simulink model "Formation_FMS2"  (R2022b)
settings: Solver=FixedStepDiscrete  StartTime=0.0  StopTime=10.0  FixedStep=FMS_CONST.dt  RelTol=1e-3
values from neighbouring files (symbols this model uses):
  FMS_PARAM = Simulink.Parameter(FMS_PARAM_VALUE)    [fms_model_init.m]
  FORMATION_PARAM = Simulink.Parameter(FORMATION_PARAM_VALUE)    [fms_model_init.m]
undefined symbols (not defined in the file or in its folder): ax_cmd, ay_cmd, CONTROL_PARAM, DiscIntNeverNeededParam, PilotMode, state, VehicleState, vh_cmd
libraries: FC_Lib x51, simulink x16
(part 1 of 3)
settings Model: Creator=19114  LastModifiedBy=19114
settings OptimizationCC: DefaultParameterBehavior=Inlined  DefaultUnderspecifiedDataType=single  EnhancedBackFolding=on  PassReuseOutputArgsAs=Individual arguments  ZeroExternalMemoryAtStartup=off  ZeroInternalMemoryAtStartup=off  MaxStackSize=64  OptimizeBlockOrder=speed  DifferentSizesBufferReuse=on  OptimizationCustomize=off  EfficientTunableParamExpr=on
settings DebuggingCC: ParameterTunabilityLossMsg=error
settings HardwareCC: ProdBitPerLong=64  ProdHWDeviceType=Intel->x86-64 (Linux 64)
settings SFSimCC: MATLABDynamicMemAlloc=off
settings RTWCC: Description=Embedded Coder  SystemTargetFile=ert.tlc  PackageGeneratedCodeAndArtifacts=on  TemplateMakefile=ert_default_tmf  TargetLang=C++
settings CodeAppCC: ForceParamTrailComments=on  IgnoreCustomStorageClasses=off  OperatorAnnotations=on  SimulinkDataObjDesc=on  SFDataObjDesc=on  InsertBlockDesc=on
settings ERTTargetCC: TargetLangStandard=C++11 (ISO)  CodeInterfacePackaging=C++ class  SupportVariableSizeSignals=on  InlinedParameterPlacement=NonHierarchical  RootIOFormat=Structure reference  ERTCustomFileTemplate=example_file_process.tlc

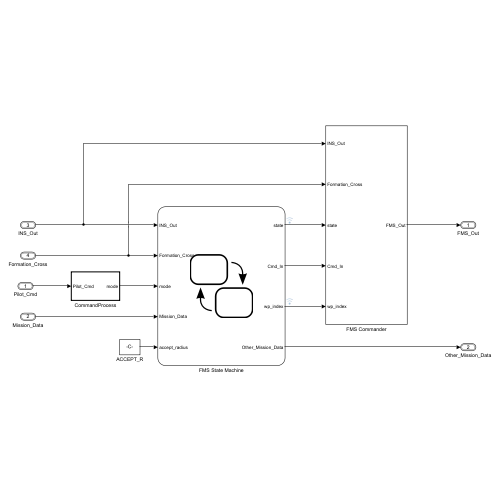
[thumbnail: Simulink's stored preview of the top-level diagram]
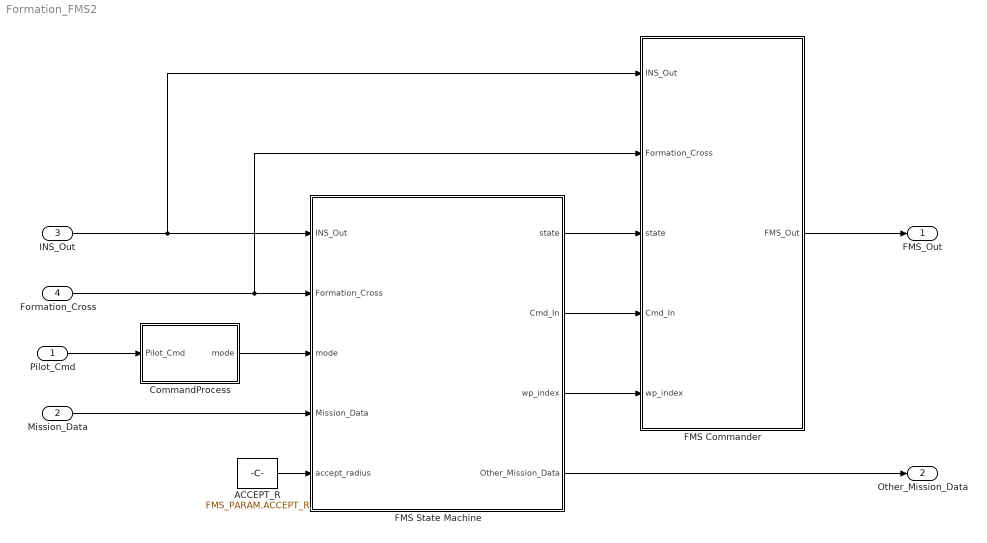
== system Formation_FMS2 ==
  Pilot_Cmd : Inport  OutDataTypeStr=Bus: Pilot_Cmd_Bus
  Mission_Data : Inport  Port=2  OutDataTypeStr=Bus: Mission_Data_Bus
  INS_Out : Inport  Port=3  OutDataTypeStr=Bus: INS_Out_Bus
  Formation_Cross : Inport  Port=4  OutDataTypeStr=Bus: Formation_Cross_Bus
  ACCEPT_R : Constant  Value=FMS_PARAM.ACCEPT_R
  CommandProcess : Subsystem  TreatAsAtomicUnit=on
  FMS Commander : Subsystem  mask{uav_id=3}
      mask DialogControl ParameterGroupVar Prompt: 参数
  FMS State Machine : Stateflow chart  TreatAsAtomicUnit=on  mask{uav_id=3, form_radius=FORMATION_PARAM.FORM_RADIUS}
  FMS_Out : Outport  OutDataTypeStr=Bus: FMS_Out_Bus  VectorParamsAs1DForOutWhenUnconnected=off
  Other_Mission_Data : Outport  Port=2  OutDataTypeStr=Bus: Other_Mission_Data_Bus  VectorParamsAs1DForOutWhenUnconnected=off
  wires:
  FMS State Machine/2(Cmd_In) -> FMS Commander/4(Cmd_In)
  ACCEPT_R/1 -> FMS State Machine/5(accept_radius)
  FMS State Machine/4(Other_Mission_Data) -> Other_Mission_Data/1
  Mission_Data/1 -> FMS State Machine/4(Mission_Data)
  Formation_Cross/1 -> FMS Commander/2(Formation_Cross), FMS State Machine/2(Formation_Cross)
  FMS State Machine/1(state) -> FMS Commander/3(state)
  CommandProcess/1(mode) -> FMS State Machine/3(mode)
  FMS Commander/1(FMS_Out) -> FMS_Out/1
  Pilot_Cmd/1 -> CommandProcess/1(Pilot_Cmd)
  FMS State Machine/3(wp_index) -> FMS Commander/5(wp_index)
  INS_Out/1 -> FMS Commander/1(INS_Out), FMS State Machine/1(INS_Out)

== system Formation_FMS2/CommandProcess ==
  Pilot_Cmd : Inport
  Check Valid : Subsystem
  Mode PreProcess : Subsystem
  mode : Outport  VectorParamsAs1DForOutWhenUnconnected=off
  wires:
  Pilot_Cmd/1 -> Check Valid/1(Pilot_Cmd), Mode PreProcess/2(Pilot_Cmd)
  Check Valid/1(pilot_cmd_valid) -> Mode PreProcess/1(pilot_cmd_valid)
  Mode PreProcess/1(mode) -> mode/1  "fms_mode"

== system Formation_FMS2/FMS Commander ==
  INS_Out : Inport
  Formation_Cross : Inport  Port=2
  state : Inport  Port=3
  Cmd_In : Inport  Port=4
  wp_index : Inport  Port=5
  Bus Creator : Subsystem
  Commander : Subsystem
  FMS_Out : Outport
  wires:
  INS_Out/1 -> Bus Creator/1(INS_Out)
  state/1 -> Bus Creator/3(state)
  Cmd_In/1 -> Bus Creator/4(Cmd_In)
  wp_index/1 -> Bus Creator/5(wp_index)
  Bus Creator/1(FMS_In) -> Commander/1(FMS_In)
  Commander/1(FMS_Out) -> FMS_Out/1
  Formation_Cross/1 -> Bus Creator/2(Formation_Cross)

== system Formation_FMS2/FMS State Machine/Vehicle.Formation.FormAssemble.dubinsPath ==
  Formation_Cross : Inport  OutDataTypeStr=Bus: Formation_Cross_Bus  PortDimensions=1
  f : TriggerPort  TriggerType=function-call  VariantControl=(inherit)
      settings: CopyFcn=Stateflow.SLINSF.SimulinkMan.removeBlockPreDeleteFcn  PreDeleteFcn=Stateflow.SLINSF.SimulinkMan.unsafePredeleteFcn
  MATLAB Function : MATLAB Function  TreatAsAtomicUnit=on  mask{form_points=FORMATION_PARAM.FORM_POINT}
  Other_Mission_Data : Outport  OutDataTypeStr=Bus: Other_Mission_Data_Bus  PortDimensions=1
  wires:
  Formation_Cross/1 -> MATLAB Function/1(ins)
  MATLAB Function/1(mission) -> Other_Mission_Data/1

== system Formation_FMS2/FMS State Machine/Vehicle.Formation.FormAssemble.dubinsPathRatio ==
  waypoints : Inport  OutDataTypeStr=single  PortDimensions=[5 5]
  pose : Inport  Port=2  OutDataTypeStr=single  PortDimensions=[1 3]
  wp_index : Inport  Port=3  OutDataTypeStr=uint16  PortDimensions=1
  f : TriggerPort  TriggerType=function-call  VariantControl=(inherit)
      settings: CopyFcn=Stateflow.SLINSF.SimulinkMan.removeBlockPreDeleteFcn  PreDeleteFcn=Stateflow.SLINSF.SimulinkMan.unsafePredeleteFcn
  Dubins Closest Point : FC_Lib/Fromation/Dubins Closest Point
      settings: LibrarySourceBlock=|
      | simulink/User-Defined
      | Functions/MATLAB Function
  Terminator : Terminator
  path_ratio : Outport  OutDataTypeStr=single  PortDimensions=1
  wires:
  Dubins Closest Point/1 -> path_ratio/1
  pose/1 -> Dubins Closest Point/2
  wp_index/1 -> Dubins Closest Point/3
  waypoints/1 -> Dubins Closest Point/1
  Dubins Closest Point/2 -> Terminator/1

== system Formation_FMS2/FMS State Machine/Vehicle.Formation.FormAssemble.testinf ==
  Input : Inport  OutDataTypeStr=single  PortDimensions=1
  f : TriggerPort  TriggerType=function-call  VariantControl=(inherit)
      settings: CopyFcn=Stateflow.SLINSF.SimulinkMan.removeBlockPreDeleteFcn  PreDeleteFcn=Stateflow.SLINSF.SimulinkMan.unsafePredeleteFcn
  MATLAB Function : MATLAB Function  TreatAsAtomicUnit=on
  Output : Outport  OutDataTypeStr=single  PortDimensions=1
  wires:
  Input/1 -> MATLAB Function/1(u)
  MATLAB Function/1(y) -> Output/1

== system Formation_FMS2/FMS State Machine/Vehicle.Formation.check_form_valid ==
  Formation_Cross : Inport  OutDataTypeStr=Bus: Formation_Cross_Bus  PortDimensions=1
  INS_Out : Inport  Port=2  OutDataTypeStr=Bus: INS_Out_Bus  PortDimensions=1
  f : TriggerPort  TriggerType=function-call  VariantControl=(inherit)
      settings: CopyFcn=Stateflow.SLINSF.SimulinkMan.removeBlockPreDeleteFcn  PreDeleteFcn=Stateflow.SLINSF.SimulinkMan.unsafePredeleteFcn
  MATLAB Function : MATLAB Function  TreatAsAtomicUnit=on  mask{form_radius=form_radius}
  valid : Outport  OutDataTypeStr=uint32  PortDimensions=1
  wires:
  Formation_Cross/1 -> MATLAB Function/1(Formation_Cross)
  INS_Out/1 -> MATLAB Function/2(INS_Out)
  MATLAB Function/1(valid) -> valid/1

== system Formation_FMS2/CommandProcess/Check Valid ==
  Pilot_Cmd : Inport
  Bus Selector1 : BusSelector  OutputSignals=timestamp
  Compare To Constant1 : simulink/Logic and Bit Operations/Compare To Constant  relop=<  const=0.5  OutDataTypeStr=boolean
  Constant1 : Constant  OutDataTypeStr=single
  Detect Change1 : simulink/Logic and Bit Operations/Detect Change  vinit=0  OutDataTypeStr=boolean
  Discrete-Time Integrator1 : DiscreteIntegrator  ExternalReset=sampled level  SampleTime=-1  SaturateOnIntegerOverflow=on  ICPrevOutput=DiscIntNeverNeededParam  ICPrevScaledInput=DiscIntNeverNeededParam
  pilot_cmd_valid : Outport  VectorParamsAs1DForOutWhenUnconnected=off
  wires:
  Pilot_Cmd/1 -> Bus Selector1/1
  Compare To Constant1/1 -> pilot_cmd_valid/1
  Bus Selector1/1 -> Detect Change1/1  "<timestamp>"
  Constant1/1 -> Discrete-Time Integrator1/1
  Detect Change1/1 -> Discrete-Time Integrator1/2
  Discrete-Time Integrator1/1 -> Compare To Constant1/1

== system Formation_FMS2/CommandProcess/Mode PreProcess ==
  pilot_cmd_valid : Inport
  Pilot_Cmd : Inport  Port=2
  Bus Selector1 : BusSelector  OutputSignals=mode
  Compare To Zero1 : simulink/Logic and Bit Operations/Compare To Zero  relop=~=  OutDataTypeStr=boolean
  Data Type Conversion2 : DataTypeConversion  OutDataTypeStr=Enum: PilotMode  SaturateOnIntegerOverflow=off  RndMeth=Floor
  Delay : Delay  DelayLength=1  InitialCondition=PilotMode.None
  Logical Operator1 : Logic  AllPortsSameDT=off  OutDataTypeStr=boolean
  Switch : Switch  Criteria=u2 > Threshold  SaturateOnIntegerOverflow=off  InputSameDT=off
  mode : Outport  VectorParamsAs1DForOutWhenUnconnected=off
  wires:
  Pilot_Cmd/1 -> Bus Selector1/1
  Bus Selector1/1 -> Compare To Zero1/1, Data Type Conversion2/1  "<mode>"
  Logical Operator1/1 -> Switch/2
  Data Type Conversion2/1 -> Switch/1
  Switch/1 -> mode/1, Delay/1
  Delay/1 -> Switch/3
  pilot_cmd_valid/1 -> Logical Operator1/2
  Compare To Zero1/1 -> Logical Operator1/1

== system Formation_FMS2/FMS Commander/Bus Creator ==
  INS_Out : Inport
  Formation_Cross : Inport  Port=2
  state : Inport  Port=3
  Cmd_In : Inport  Port=4
  wp_index : Inport  Port=5
  Bus Creator : BusCreator  Inputs=5
  Signal Copy{1..3,5..6} (5 alike) : SignalConversion  OverrideOpt=off
  FMS_In : Outport
  wires:
  Bus Creator/1 -> FMS_In/1
  wp_index/1 -> Signal Copy5/1
  Signal Copy3/1 -> Bus Creator/4  "Cmd_In"
  Signal Copy1/1 -> Bus Creator/1  "INS_Out"
  INS_Out/1 -> Signal Copy1/1
  Signal Copy5/1 -> Bus Creator/5  "wp_index"
  Signal Copy6/1 -> Bus Creator/3  "vehicle_state"
  state/1 -> Signal Copy6/1
  Cmd_In/1 -> Signal Copy3/1
  Formation_Cross/1 -> Signal Copy2/1
  Signal Copy2/1 -> Bus Creator/2  "Formation_Cross"

== system Formation_FMS2/FMS Commander/Commander ==
  FMS_In : Inport
  Bus Selector : BusSelector  OutputSignals=vehicle_state
  Default : Subsystem
      settings: UndoDeleteFcn=Stateflow.SLINSF.SimulinkMan.restorePreDeleteFcn  PreDeleteFcn=Stateflow.SLINSF.SimulinkMan.removePreDeleteFcn
  FMS_In1 : InportShadow
  FMS_In2 : InportShadow
  FMS_In3 : InportShadow
  Form_Subsystem : Subsystem  TreatAsAtomicUnit=on
  Hold : Subsystem
      settings: UndoDeleteFcn=Stateflow.SLINSF.SimulinkMan.restorePreDeleteFcn  PreDeleteFcn=Stateflow.SLINSF.SimulinkMan.removePreDeleteFcn
  Merge : Merge  Inputs=3
  Switch Case : SwitchCase  CaseConditions={[VehicleState.FormAssemble,VehicleState.FormHold,VehicleState.FormMission,VehicleState.FormDisband],VehicleState.Hold}
  FMS_Out : Outport
  wires:
  FMS_In/1 -> Bus Selector/1
  Bus Selector/1 -> Switch Case/1  "<vehicle_state>"
  Switch Case/1 -> Form_Subsystem/Action
  FMS_In1/1 -> Form_Subsystem/1(FMS_In)
  Form_Subsystem/1(FMS_Out) -> Merge/1
  Merge/1 -> FMS_Out/1
  Switch Case/2 -> Hold/Action
  Hold/1(FMS_Out) -> Merge/2
  FMS_In2/1 -> Hold/1(FMS_In)
  Switch Case/3 -> Default/Action
  Default/1(FMS_Out) -> Merge/3
  FMS_In3/1 -> Default/1(FMS_In)

== system Formation_FMS2/FMS Commander/Commander/Default ==
  FMS_In : Inport
  Action Port : ActionPort  InitializeStates=reset
      settings: CopyFcn=Stateflow.SLINSF.SimulinkMan.removeBlockPreDeleteFcn
  Airspeed Hold : Subsystem
  Altitude_Hold : Subsystem
  Bus Assignment : BusAssignment  AssignedSignals=state,ax_cmd,ay_cmd,vh_cmd
  Constant : Constant  Value=0  OutDataTypeStr=Bus: FMS_Out_Bus
  Constant1 : Constant  Value=VehicleState.None  OutDataTypeStr=Enum: VehicleState
  Loiter_Control : Subsystem  Commented=on
  FMS_Out : Outport  VectorParamsAs1DForOutWhenUnconnected=off
  wires:
  Airspeed Hold/1(ax_cmd) -> Bus Assignment/3
  Loiter_Control/1(ay_cmd_mPs2) -> Bus Assignment/4
  FMS_In/1 -> Airspeed Hold/1(FMS_In), Altitude_Hold/1(FMS_In), Loiter_Control/1(FMS_In)
  Constant/1 -> Bus Assignment/1
  Altitude_Hold/1(vh_cmd_mPs) -> Bus Assignment/5
  Bus Assignment/1 -> FMS_Out/1
  Constant1/1 -> Bus Assignment/2

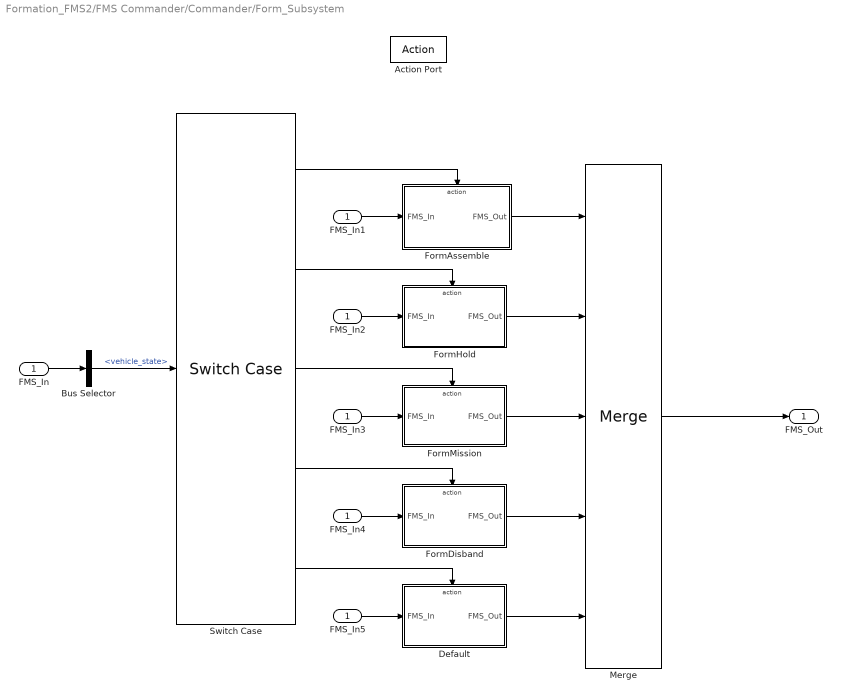
== system Formation_FMS2/FMS Commander/Commander/Form_Subsystem ==
  FMS_In : Inport
  Action Port : ActionPort
  Bus Selector : BusSelector  OutputSignals=vehicle_state
  Default : Subsystem
      settings: UndoDeleteFcn=Stateflow.SLINSF.SimulinkMan.restorePreDeleteFcn  PreDeleteFcn=Stateflow.SLINSF.SimulinkMan.removePreDeleteFcn
  FMS_In{1..5} (5 alike) : InportShadow
  FormAssemble : Subsystem  TreatAsAtomicUnit=on
  FormDisband : Subsystem
      settings: UndoDeleteFcn=Stateflow.SLINSF.SimulinkMan.restorePreDeleteFcn  PreDeleteFcn=Stateflow.SLINSF.SimulinkMan.removePreDeleteFcn
  FormHold : Subsystem
      settings: UndoDeleteFcn=Stateflow.SLINSF.SimulinkMan.restorePreDeleteFcn  PreDeleteFcn=Stateflow.SLINSF.SimulinkMan.removePreDeleteFcn
  FormMission : Subsystem  TreatAsAtomicUnit=on
  Merge : Merge  Inputs=5
  Switch Case : SwitchCase  CaseConditions={VehicleState.FormAssemble,VehicleState.FormHold,VehicleState.FormMission,VehicleState.FormDisband}
  FMS_Out : Outport
  wires:
  Merge/1 -> FMS_Out/1
  FMS_In/1 -> Bus Selector/1
  Bus Selector/1 -> Switch Case/1  "<vehicle_state>"
  Switch Case/5 -> Default/Action
  Default/1(FMS_Out) -> Merge/5
  Switch Case/3 -> FormMission/Action
  FMS_In1/1 -> FormAssemble/1(FMS_In)
  Switch Case/1 -> FormAssemble/Action
  FMS_In2/1 -> FormHold/1(FMS_In)
  Switch Case/2 -> FormHold/Action
  FMS_In3/1 -> FormMission/1(FMS_In)
  Switch Case/4 -> FormDisband/Action
  FMS_In4/1 -> FormDisband/1(FMS_In)
  FMS_In5/1 -> Default/1(FMS_In)
  FormAssemble/1(FMS_Out) -> Merge/1
  FormHold/1(FMS_Out) -> Merge/2
  FormMission/1(FMS_Out) -> Merge/3
  FormDisband/1(FMS_Out) -> Merge/4

== system Formation_FMS2/FMS Commander/Commander/Hold ==
  FMS_In : Inport
  Action Port : ActionPort  InitializeStates=reset
      settings: CopyFcn=Stateflow.SLINSF.SimulinkMan.removeBlockPreDeleteFcn
  Airspeed Hold : Subsystem
  Altitude_Hold : Subsystem
  Bus Assignment : BusAssignment  AssignedSignals=state,ax_cmd,ay_cmd,vh_cmd
  Constant : Constant  Value=0  OutDataTypeStr=Bus: FMS_Out_Bus
  Constant1 : Constant  Value=VehicleState.Hold  OutDataTypeStr=Enum: VehicleState
  Loiter_Control : Subsystem
  FMS_Out : Outport  VectorParamsAs1DForOutWhenUnconnected=off
  wires:
  Bus Assignment/1 -> FMS_Out/1
  Altitude_Hold/1(vh_cmd_mPs) -> Bus Assignment/5
  Constant/1 -> Bus Assignment/1
  FMS_In/1 -> Altitude_Hold/1(FMS_In), Airspeed Hold/1(FMS_In), Loiter_Control/1(FMS_In)
  Loiter_Control/1(ay_cmd_mPs2) -> Bus Assignment/4
  Airspeed Hold/1(ax_cmd) -> Bus Assignment/3
  Constant1/1 -> Bus Assignment/2

== system Formation_FMS2/FMS Commander/Commander/Default/Airspeed Hold ==
  FMS_In : Inport
  Bus Selector : BusSelector  OutputSignals=INS_Out.airspeed
  Constant : Constant  Value=FMS_PARAM.FW_AIRSPD_TRIM
  Gain : Gain
  Sum : Sum  Inputs=-+|
  ax_cmd : Outport
  wires:
  Bus Selector/1 -> Sum/1  "<airspeed>"
  FMS_In/1 -> Bus Selector/1
  Constant/1 -> Sum/2
  Gain/1 -> ax_cmd/1  "ax_cmd"
  Sum/1 -> Gain/1  "v_error"

== system Formation_FMS2/FMS Commander/Commander/Default/Altitude_Hold ==
  FMS_In : Inport
  Bus Selector2 : BusSelector  OutputSignals=INS_Out.h_R
  Delay : Delay  DelayLength=1  InitialConditionSource=Input port
      settings: InputPortMap=u0,p4
  Gain2 : Gain  Gain=FMS_PARAM.Z_P  OutDataTypeStr=single
  Saturation : Saturate  UpperLimit=CONTROL_PARAM.FW_T_CLMB_MAX  LowerLimit=-CONTROL_PARAM.FW_T_SINK_MAX
  Sum : Sum  Inputs=-+|
  vh_cmd_mPs : Outport  VectorParamsAs1DForOutWhenUnconnected=off
  wires:
  Gain2/1 -> Saturation/1
  Bus Selector2/1 -> Delay/2, Sum/1  "<h_R>"
  Sum/1 -> Gain2/1  "h_err_R"
  Delay/1 -> Sum/2, Delay/1  "h_cmd_R"
  FMS_In/1 -> Bus Selector2/1
  Saturation/1 -> vh_cmd_mPs/1

== system Formation_FMS2/FMS Commander/Commander/Default/Loiter_Control ==
  FMS_In : Inport
  Bus Selector2 : BusSelector  OutputSignals=INS_Out.vn,INS_Out.ve
  L1 : Constant  Value=FMS_PARAM.L1  OutDataTypeStr=single
  L1 Reference WP : Subsystem
  L1_Core : Subsystem
  Mux1 : Mux  Inputs=2
  R : Constant  Value=FMS_PARAM.LOITER_R  OutDataTypeStr=single
  Reference_Point : Subsystem
  ay_cmd_mPs2 : Outport  VectorParamsAs1DForOutWhenUnconnected=off
  wires:
  Mux1/1 -> L1_Core/4(Vg)
  Bus Selector2/1 -> Mux1/1  "<vn>"
  Bus Selector2/2 -> Mux1/2  "<ve>"
  FMS_In/1 -> Reference_Point/1(FMS_In), Bus Selector2/1
  L1/1 -> L1 Reference WP/5(L1), L1_Core/3(L1)
  R/1 -> L1 Reference WP/4(R)
  Reference_Point/3(n) -> L1 Reference WP/3(n)
  Reference_Point/2(p_0) -> L1 Reference WP/2(P_0)
  Reference_Point/1(p_vehicle) -> L1 Reference WP/1(P_Vehicle), L1_Core/1(p_vehicle)
  L1_Core/1(ay_cmd_mPs2) -> ay_cmd_mPs2/1
  L1 Reference WP/1(L1_WP) -> L1_Core/2(L1_WP)  "L1_WP"

== system Formation_FMS2/FMS Commander/Commander/Form_Subsystem/Default ==
  FMS_In : Inport
  Action Port : ActionPort  InitializeStates=reset
      settings: CopyFcn=Stateflow.SLINSF.SimulinkMan.removeBlockPreDeleteFcn
  Airspeed Hold : Subsystem
  Altitude_Hold : Subsystem
  Bus Assignment : BusAssignment  AssignedSignals=state,ax_cmd,ay_cmd,vh_cmd
  Constant : Constant  Value=0  OutDataTypeStr=Bus: FMS_Out_Bus
  Constant1 : Constant  Value=VehicleState.None  OutDataTypeStr=Enum: VehicleState
  Loiter_Control : Subsystem  Commented=on
  FMS_Out : Outport  VectorParamsAs1DForOutWhenUnconnected=off
  wires:
  Airspeed Hold/1(ax_cmd) -> Bus Assignment/3
  Loiter_Control/1(ay_cmd_mPs2) -> Bus Assignment/4
  FMS_In/1 -> Airspeed Hold/1(FMS_In), Altitude_Hold/1(FMS_In), Loiter_Control/1(FMS_In)
  Constant/1 -> Bus Assignment/1
  Altitude_Hold/1(vh_cmd_mPs) -> Bus Assignment/5
  Bus Assignment/1 -> FMS_Out/1
  Constant1/1 -> Bus Assignment/2

== system Formation_FMS2/FMS Commander/Commander/Form_Subsystem/FormAssemble ==
  FMS_In : Inport
  Action Port : ActionPort
  Bus Selector : BusSelector  OutputSignals=wp_index
  Detect Change : simulink/Logic and Bit Operations/Detect Change  vinit=0  OutDataTypeStr=boolean
  Mission_SubSystem : Subsystem  TreatAsAtomicUnit=on
  FMS_Out : Outport
  wires:
  FMS_In/1 -> Bus Selector/1, Mission_SubSystem/1(FMS_In)
  Mission_SubSystem/1(FMS_Out) -> FMS_Out/1
  Detect Change/1 -> Mission_SubSystem/Reset
  Bus Selector/1 -> Detect Change/1  "<wp_index>"

== system Formation_FMS2/FMS Commander/Commander/Form_Subsystem/FormDisband ==
  FMS_In : Inport
  Action Port : ActionPort  InitializeStates=reset
      settings: CopyFcn=Stateflow.SLINSF.SimulinkMan.removeBlockPreDeleteFcn
  Airspeed Hold : Subsystem
  Altitude_Hold : Subsystem
  Bus Assignment : BusAssignment  AssignedSignals=state,ax_cmd,ay_cmd,vh_cmd
  Constant : Constant  Value=0  OutDataTypeStr=Bus: FMS_Out_Bus
  Constant1 : Constant  Value=VehicleState.FormDisband  OutDataTypeStr=Enum: VehicleState
  Loiter_Control : Subsystem
  FMS_Out : Outport  VectorParamsAs1DForOutWhenUnconnected=off
  wires:
  Constant1/1 -> Bus Assignment/2
  Airspeed Hold/1(ax_cmd) -> Bus Assignment/3
  Loiter_Control/1(ay_cmd_mPs2) -> Bus Assignment/4
  FMS_In/1 -> Loiter_Control/1(FMS_In), Airspeed Hold/1(FMS_In), Altitude_Hold/1(FMS_In)
  Constant/1 -> Bus Assignment/1
  Altitude_Hold/1(vh_cmd_mPs) -> Bus Assignment/5
  Bus Assignment/1 -> FMS_Out/1

== system Formation_FMS2/FMS Commander/Commander/Form_Subsystem/FormHold ==
  FMS_In : Inport
  Action Port : ActionPort  InitializeStates=reset
      settings: CopyFcn=Stateflow.SLINSF.SimulinkMan.removeBlockPreDeleteFcn
  Airspeed Hold : Subsystem
  Altitude_Hold : Subsystem
  Bus Assignment : BusAssignment  AssignedSignals=state,ax_cmd,ay_cmd,vh_cmd
  Constant : Constant  Value=0  OutDataTypeStr=Bus: FMS_Out_Bus
  Constant1 : Constant  Value=VehicleState.FormHold  OutDataTypeStr=Enum: VehicleState
  Loiter_Control : Subsystem
  FMS_Out : Outport  VectorParamsAs1DForOutWhenUnconnected=off
  wires:
  Bus Assignment/1 -> FMS_Out/1
  Altitude_Hold/1(vh_cmd_mPs) -> Bus Assignment/5
  Constant/1 -> Bus Assignment/1
  FMS_In/1 -> Altitude_Hold/1(FMS_In), Airspeed Hold/1(FMS_In), Loiter_Control/1(FMS_In)
  Loiter_Control/1(ay_cmd_mPs2) -> Bus Assignment/4
  Airspeed Hold/1(ax_cmd) -> Bus Assignment/3
  Constant1/1 -> Bus Assignment/2

== system Formation_FMS2/FMS Commander/Commander/Form_Subsystem/FormMission ==
  FMS_In : Inport
  Action Port : ActionPort
  Bus Selector : BusSelector  OutputSignals=wp_index
  Detect Change : simulink/Logic and Bit Operations/Detect Change  vinit=0  OutDataTypeStr=boolean
  FormMission_SubSystem : Subsystem  TreatAsAtomicUnit=on
  FMS_Out : Outport
  wires:
  FMS_In/1 -> Bus Selector/1, FormMission_SubSystem/1(FMS_In)
  FormMission_SubSystem/1(FMS_Out) -> FMS_Out/1
  Detect Change/1 -> FormMission_SubSystem/Reset
  Bus Selector/1 -> Detect Change/1  "<wp_index>"

== system Formation_FMS2/FMS Commander/Commander/Hold/Airspeed Hold ==
  FMS_In : Inport
  Bus Selector : BusSelector  OutputSignals=INS_Out.airspeed
  Constant : Constant  Value=FMS_PARAM.FW_AIRSPD_TRIM
  Gain : Gain
  Sum : Sum  Inputs=-+|
  ax_cmd : Outport
  wires:
  Sum/1 -> Gain/1  "v_error"
  Gain/1 -> ax_cmd/1  "ax_cmd"
  Constant/1 -> Sum/2
  FMS_In/1 -> Bus Selector/1
  Bus Selector/1 -> Sum/1  "<airspeed>"

== system Formation_FMS2/FMS Commander/Commander/Hold/Altitude_Hold ==
  FMS_In : Inport
  Bus Selector2 : BusSelector  OutputSignals=INS_Out.h_R
  Constant : Constant  Value=FMS_PARAM.FW_HEIGHT_TRIM
  Delay : Delay  DelayLength=1  InitialConditionSource=Input port
      settings: InputPortMap=u0,p4
  Gain2 : Gain  Gain=FMS_PARAM.Z_P  OutDataTypeStr=single
  Saturation : Saturate  UpperLimit=CONTROL_PARAM.FW_T_CLMB_MAX  LowerLimit=-CONTROL_PARAM.FW_T_SINK_MAX
  Sum : Sum  Inputs=-+|
  vh_cmd_mPs : Outport  VectorParamsAs1DForOutWhenUnconnected=off
  wires:
  Gain2/1 -> Saturation/1
  Bus Selector2/1 -> Sum/1  "<h_R>"
  Sum/1 -> Gain2/1  "h_err_R"
  Delay/1 -> Sum/2, Delay/1  "h_cmd_R"
  FMS_In/1 -> Bus Selector2/1
  Saturation/1 -> vh_cmd_mPs/1
  Constant/1 -> Delay/2

== system Formation_FMS2/FMS Commander/Commander/Hold/Loiter_Control ==
  FMS_In : Inport
  Bus Selector2 : BusSelector  OutputSignals=INS_Out.vn,INS_Out.ve
  L1 : Constant  Value=FMS_PARAM.L1  OutDataTypeStr=single
  L1 Reference WP : Subsystem
  L1_Core : Subsystem
  Mux1 : Mux  Inputs=2
  R : Constant  Value=FMS_PARAM.LOITER_R  OutDataTypeStr=single
  Reference_Point : Subsystem
  ay_cmd_mPs2 : Outport  VectorParamsAs1DForOutWhenUnconnected=off
  wires:
  L1 Reference WP/1(L1_WP) -> L1_Core/2(L1_WP)  "L1_WP"
  L1_Core/1(ay_cmd_mPs2) -> ay_cmd_mPs2/1
  Reference_Point/1(p_vehicle) -> L1_Core/1(p_vehicle), L1 Reference WP/1(P_Vehicle)
  Reference_Point/2(p_0) -> L1 Reference WP/2(P_0)
  Reference_Point/3(n) -> L1 Reference WP/3(n)
  R/1 -> L1 Reference WP/4(R)
  L1/1 -> L1_Core/3(L1), L1 Reference WP/5(L1)
  FMS_In/1 -> Bus Selector2/1, Reference_Point/1(FMS_In)
  Bus Selector2/2 -> Mux1/2  "<ve>"
  Bus Selector2/1 -> Mux1/1  "<vn>"
  Mux1/1 -> L1_Core/4(Vg)

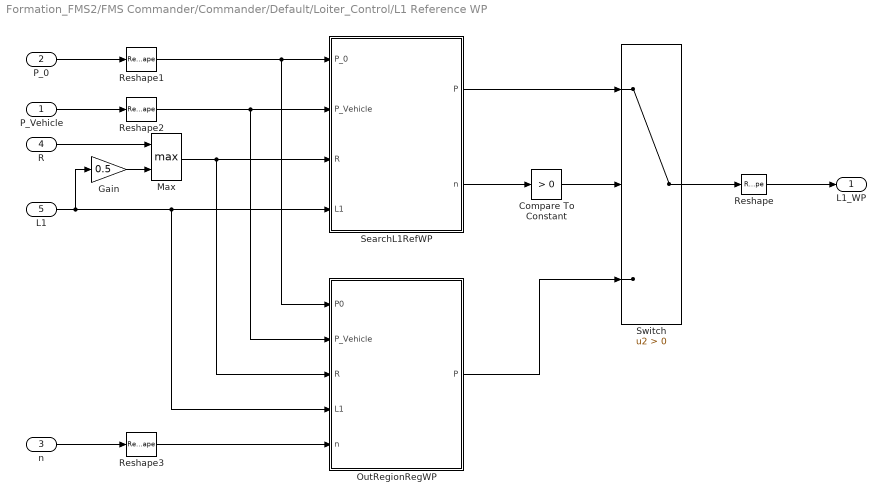
== system Formation_FMS2/FMS Commander/Commander/Default/Loiter_Control/L1 Reference WP ==
  P_Vehicle : Inport
  P_0 : Inport  Port=2
  n : Inport  Port=3
  R : Inport  Port=4
  L1 : Inport  Port=5
  Compare To Constant : simulink/Logic and Bit Operations/Compare To Constant  relop=>  const=0  OutDataTypeStr=boolean
  Gain : Gain  Gain=0.5
  Max : MinMax  Function=max  Inputs=2
  OutRegionRegWP : MATLAB Function  TreatAsAtomicUnit=on
  Reshape : Reshape  OutputDimensionality=Customize  OutputDimensions=[2,1]
  Reshape1 : Reshape  OutputDimensionality=Column vector (2-D)
  Reshape2 : Reshape  OutputDimensionality=Column vector (2-D)
  Reshape3 : Reshape  OutputDimensionality=Column vector (2-D)
  SearchL1RefWP : MATLAB Function  TreatAsAtomicUnit=on
  Switch : Switch  Criteria=u2 > Threshold  SaturateOnIntegerOverflow=off  InputSameDT=off
  L1_WP : Outport  VectorParamsAs1DForOutWhenUnconnected=off
  wires:
  Gain/1 -> Max/2
  R/1 -> Max/1
  Reshape3/1 -> OutRegionRegWP/5(n)
  n/1 -> Reshape3/1
  Reshape2/1 -> SearchL1RefWP/2(P_Vehicle), OutRegionRegWP/2(P_Vehicle)
  Reshape1/1 -> SearchL1RefWP/1(P_0), OutRegionRegWP/1(P0)
  L1/1 -> SearchL1RefWP/4(L1), OutRegionRegWP/4(L1), Gain/1
  Max/1 -> SearchL1RefWP/3(R), OutRegionRegWP/3(R)
  P_Vehicle/1 -> Reshape2/1
  P_0/1 -> Reshape1/1
  SearchL1RefWP/1(P) -> Switch/1
  Switch/1 -> Reshape/1
  OutRegionRegWP/1(P) -> Switch/3
  SearchL1RefWP/2(n) -> Compare To Constant/1
  Compare To Constant/1 -> Switch/2
  Reshape/1 -> L1_WP/1

== system Formation_FMS2/FMS Commander/Commander/Default/Loiter_Control/L1_Core ==
  p_vehicle : Inport
  L1_WP : Inport  Port=2
  L1 : Inport  Port=3
  Vg : Inport  Port=4
  L1_Lateral_Acceleration : Subsystem
  Subtract : Sum  Inputs=+-
  ay_cmd_mPs2 : Outport  VectorParamsAs1DForOutWhenUnconnected=off
  wires:
  L1_Lateral_Acceleration/1(l1_a_cmd) -> ay_cmd_mPs2/1
  Subtract/1 -> L1_Lateral_Acceleration/3(l1_path)
  Vg/1 -> L1_Lateral_Acceleration/2(Vg)
  L1/1 -> L1_Lateral_Acceleration/1(L1)
  p_vehicle/1 -> Subtract/2
  L1_WP/1 -> Subtract/1

== system Formation_FMS2/FMS Commander/Commander/Default/Loiter_Control/Reference_Point ==
  FMS_In : Inport
  Bus Selector1 : BusSelector  OutputSignals=Cmd_In.cur_waypoint
  Bus Selector2 : BusSelector  OutputSignals=INS_Out.vn,INS_Out.ve
  Bus Selector3 : BusSelector  OutputSignals=INS_Out.x_R,INS_Out.y_R
  Mux1 : Mux  Inputs=2
  Mux2 : Mux  Inputs=2
  Selector : Selector  InputPortWidth=3  IndexOptions=Index vector (dialog)  Indices=[1 2]  OutputSizes=1
  Vector Normalize : FC_Lib/Math/Vector Normalize
      settings: SourceProductName=Flight Control Toolbox
  start_vel : Delay  DelayLength=1  InitialConditionSource=Input port
      settings: InputPortMap=u0,p4
  p_vehicle : Outport  VectorParamsAs1DForOutWhenUnconnected=off
  p_0 : Outport  Port=2  VectorParamsAs1DForOutWhenUnconnected=off
  n : Outport  Port=3  VectorParamsAs1DForOutWhenUnconnected=off
  wires:
  Selector/1 -> p_0/1
  Bus Selector1/1 -> Selector/1  "<cur_waypoint>"
  Mux2/1 -> p_vehicle/1
  Bus Selector3/2 -> Mux2/2  "<y_R>"
  Bus Selector3/1 -> Mux2/1  "<x_R>"
  Mux1/1 -> start_vel/2
  FMS_In/1 -> Bus Selector1/1, Bus Selector2/1, Bus Selector3/1
  Vector Normalize/1 -> n/1
  Bus Selector2/1 -> Mux1/1  "<vn>"
  start_vel/1 -> start_vel/1, Vector Normalize/1
  Bus Selector2/2 -> Mux1/2  "<ve>"

== system Formation_FMS2/FMS Commander/Commander/Form_Subsystem/Default/Airspeed Hold ==
  FMS_In : Inport
  Bus Selector : BusSelector  OutputSignals=INS_Out.airspeed
  Constant : Constant  Value=FMS_PARAM.FW_AIRSPD_TRIM
  Gain : Gain
  Sum : Sum  Inputs=-+|
  ax_cmd : Outport
  wires:
  Bus Selector/1 -> Sum/1  "<airspeed>"
  FMS_In/1 -> Bus Selector/1
  Constant/1 -> Sum/2
  Gain/1 -> ax_cmd/1  "ax_cmd"
  Sum/1 -> Gain/1  "v_error"

== system Formation_FMS2/FMS Commander/Commander/Form_Subsystem/Default/Altitude_Hold ==
  FMS_In : Inport
  Bus Selector2 : BusSelector  OutputSignals=INS_Out.h_R
  Delay : Delay  DelayLength=1  InitialConditionSource=Input port
      settings: InputPortMap=u0,p4
  Gain2 : Gain  Gain=FMS_PARAM.Z_P  OutDataTypeStr=single
  Saturation : Saturate  UpperLimit=CONTROL_PARAM.FW_T_CLMB_MAX  LowerLimit=-CONTROL_PARAM.FW_T_SINK_MAX
  Sum : Sum  Inputs=-+|
  vh_cmd_mPs : Outport  VectorParamsAs1DForOutWhenUnconnected=off
  wires:
  Gain2/1 -> Saturation/1
  Bus Selector2/1 -> Delay/2, Sum/1  "<h_R>"
  Sum/1 -> Gain2/1  "h_err_R"
  Delay/1 -> Sum/2, Delay/1  "h_cmd_R"
  FMS_In/1 -> Bus Selector2/1
  Saturation/1 -> vh_cmd_mPs/1

== system Formation_FMS2/FMS Commander/Commander/Form_Subsystem/Default/Loiter_Control ==
  FMS_In : Inport
  Bus Selector2 : BusSelector  OutputSignals=INS_Out.vn,INS_Out.ve
  L1 : Constant  Value=FMS_PARAM.L1  OutDataTypeStr=single
  L1 Reference WP : Subsystem
  L1_Core : Subsystem
  Mux1 : Mux  Inputs=2
  R : Constant  Value=FMS_PARAM.LOITER_R  OutDataTypeStr=single
  Reference_Point : Subsystem
  ay_cmd_mPs2 : Outport  VectorParamsAs1DForOutWhenUnconnected=off
  wires:
  Mux1/1 -> L1_Core/4(Vg)
  Bus Selector2/1 -> Mux1/1  "<vn>"
  Bus Selector2/2 -> Mux1/2  "<ve>"
  FMS_In/1 -> Reference_Point/1(FMS_In), Bus Selector2/1
  L1/1 -> L1 Reference WP/5(L1), L1_Core/3(L1)
  R/1 -> L1 Reference WP/4(R)
  Reference_Point/3(n) -> L1 Reference WP/3(n)
  Reference_Point/2(p_0) -> L1 Reference WP/2(P_0)
  Reference_Point/1(p_vehicle) -> L1 Reference WP/1(P_Vehicle), L1_Core/1(p_vehicle)
  L1_Core/1(ay_cmd_mPs2) -> ay_cmd_mPs2/1
  L1 Reference WP/1(L1_WP) -> L1_Core/2(L1_WP)  "L1_WP"

== system Formation_FMS2/FMS Commander/Commander/Form_Subsystem/FormAssemble/Mission_SubSystem ==
  FMS_In : Inport
  Reset : ResetPort  DisableCoverage=on
  Airspeed Hold : Subsystem
  Altitude Control : Subsystem  Commented=on
  Altitude_Hold : Subsystem
  Bus Assignment : BusAssignment  AssignedSignals=state,ax_cmd,ay_cmd,vh_cmd
  Constant : Constant  Value=0  OutDataTypeStr=Bus: FMS_Out_Bus
  Constant1 : Constant  Value=VehicleState.FormAssemble  OutDataTypeStr=Enum: VehicleState
  Position Command : Subsystem
  testnan : MATLAB Function  Commented=on  TreatAsAtomicUnit=on
  FMS_Out : Outport  VectorParamsAs1DForOutWhenUnconnected=off
  wires:
  Constant/1 -> Bus Assignment/1
  Bus Assignment/1 -> FMS_Out/1
  Position Command/1(ay_cmd_mPs2) -> Bus Assignment/4
  Altitude_Hold/1(vh_cmd_mPs) -> Bus Assignment/5
  Airspeed Hold/1(ax_cmd) -> Bus Assignment/3
  Constant1/1 -> Bus Assignment/2
  FMS_In/1 -> Airspeed Hold/1(FMS_In), Position Command/1(FMS_In), Altitude_Hold/1(FMS_In)

== system Formation_FMS2/FMS Commander/Commander/Form_Subsystem/FormDisband/Airspeed Hold ==
  FMS_In : Inport
  Bus Selector : BusSelector  OutputSignals=INS_Out.airspeed
  Constant : Constant  Value=FMS_PARAM.FW_AIRSPD_TRIM
  Gain : Gain
  Sum : Sum  Inputs=-+|
  ax_cmd : Outport
  wires:
  Bus Selector/1 -> Sum/1  "<airspeed>"
  FMS_In/1 -> Bus Selector/1
  Constant/1 -> Sum/2
  Gain/1 -> ax_cmd/1  "ax_cmd"
  Sum/1 -> Gain/1  "v_error"

== system Formation_FMS2/FMS Commander/Commander/Form_Subsystem/FormDisband/Altitude_Hold ==
  FMS_In : Inport
  Bus Selector2 : BusSelector  OutputSignals=INS_Out.h_R
  Constant : Constant  Value=FMS_PARAM.FW_HEIGHT_TRIM
  Delay : Delay  DelayLength=1  InitialConditionSource=Input port
      settings: InputPortMap=u0,p4
  Gain2 : Gain  Gain=FMS_PARAM.Z_P  OutDataTypeStr=single
  Saturation : Saturate  UpperLimit=CONTROL_PARAM.FW_T_CLMB_MAX  LowerLimit=-CONTROL_PARAM.FW_T_SINK_MAX
  Sum : Sum  Inputs=-+|
  vh_cmd_mPs : Outport  VectorParamsAs1DForOutWhenUnconnected=off
  wires:
  Constant/1 -> Delay/2
  Saturation/1 -> vh_cmd_mPs/1
  FMS_In/1 -> Bus Selector2/1
  Delay/1 -> Delay/1, Sum/2  "h_cmd_R"
  Sum/1 -> Gain2/1  "h_err_R"
  Bus Selector2/1 -> Sum/1  "<h_R>"
  Gain2/1 -> Saturation/1

== system Formation_FMS2/FMS Commander/Commander/Form_Subsystem/FormDisband/Loiter_Control ==
  FMS_In : Inport
  Bus Selector2 : BusSelector  OutputSignals=INS_Out.vn,INS_Out.ve
  L1 : Constant  Value=FMS_PARAM.L1  OutDataTypeStr=single
  L1 Reference WP : Subsystem
  L1_Core : Subsystem
  Mux1 : Mux  Inputs=2
  R : Constant  Value=FMS_PARAM.LOITER_R  OutDataTypeStr=single
  Reference_Point : Subsystem
  ay_cmd_mPs2 : Outport  VectorParamsAs1DForOutWhenUnconnected=off
  wires:
  Mux1/1 -> L1_Core/4(Vg)
  Bus Selector2/1 -> Mux1/1  "<vn>"
  Bus Selector2/2 -> Mux1/2  "<ve>"
  FMS_In/1 -> Reference_Point/1(FMS_In), Bus Selector2/1
  L1/1 -> L1 Reference WP/5(L1), L1_Core/3(L1)
  R/1 -> L1 Reference WP/4(R)
  Reference_Point/3(n) -> L1 Reference WP/3(n)
  Reference_Point/2(p_0) -> L1 Reference WP/2(P_0)
  Reference_Point/1(p_vehicle) -> L1 Reference WP/1(P_Vehicle), L1_Core/1(p_vehicle)
  L1_Core/1(ay_cmd_mPs2) -> ay_cmd_mPs2/1
  L1 Reference WP/1(L1_WP) -> L1_Core/2(L1_WP)  "L1_WP"

== system Formation_FMS2/FMS Commander/Commander/Form_Subsystem/FormHold/Airspeed Hold ==
  FMS_In : Inport
  Bus Selector : BusSelector  OutputSignals=INS_Out.airspeed
  Constant : Constant  Value=FMS_PARAM.FW_AIRSPD_TRIM
  Gain : Gain
  Sum : Sum  Inputs=-+|
  ax_cmd : Outport
  wires:
  Sum/1 -> Gain/1  "v_error"
  Gain/1 -> ax_cmd/1  "ax_cmd"
  Constant/1 -> Sum/2
  FMS_In/1 -> Bus Selector/1
  Bus Selector/1 -> Sum/1  "<airspeed>"

== system Formation_FMS2/FMS Commander/Commander/Form_Subsystem/FormHold/Altitude_Hold ==
  FMS_In : Inport
  Bus Selector2 : BusSelector  OutputSignals=INS_Out.h_R
  Constant : Constant  Value=FMS_PARAM.FW_HEIGHT_TRIM
  Delay : Delay  DelayLength=1  InitialConditionSource=Input port
      settings: InputPortMap=u0,p4
  Gain2 : Gain  Gain=FMS_PARAM.Z_P  OutDataTypeStr=single
  Saturation : Saturate  UpperLimit=CONTROL_PARAM.FW_T_CLMB_MAX  LowerLimit=-CONTROL_PARAM.FW_T_SINK_MAX
  Sum : Sum  Inputs=-+|
  vh_cmd_mPs : Outport  VectorParamsAs1DForOutWhenUnconnected=off
  wires:
  Gain2/1 -> Saturation/1
  Bus Selector2/1 -> Sum/1  "<h_R>"
  Sum/1 -> Gain2/1  "h_err_R"
  Delay/1 -> Sum/2, Delay/1  "h_cmd_R"
  FMS_In/1 -> Bus Selector2/1
  Saturation/1 -> vh_cmd_mPs/1
  Constant/1 -> Delay/2

== system Formation_FMS2/FMS Commander/Commander/Form_Subsystem/FormHold/Loiter_Control ==
  FMS_In : Inport
  Bus Selector2 : BusSelector  OutputSignals=INS_Out.vn,INS_Out.ve
  L1 : Constant  Value=FMS_PARAM.L1  OutDataTypeStr=single
  L1 Reference WP : Subsystem
  L1_Core : Subsystem
  Mux1 : Mux  Inputs=2
  R : Constant  Value=FMS_PARAM.LOITER_R  OutDataTypeStr=single
  Reference_Point : Subsystem
  ay_cmd_mPs2 : Outport  VectorParamsAs1DForOutWhenUnconnected=off
  wires:
  L1 Reference WP/1(L1_WP) -> L1_Core/2(L1_WP)  "L1_WP"
  L1_Core/1(ay_cmd_mPs2) -> ay_cmd_mPs2/1
  Reference_Point/1(p_vehicle) -> L1_Core/1(p_vehicle), L1 Reference WP/1(P_Vehicle)
  Reference_Point/2(p_0) -> L1 Reference WP/2(P_0)
  Reference_Point/3(n) -> L1 Reference WP/3(n)
  R/1 -> L1 Reference WP/4(R)
  L1/1 -> L1_Core/3(L1), L1 Reference WP/5(L1)
  FMS_In/1 -> Bus Selector2/1, Reference_Point/1(FMS_In)
  Bus Selector2/2 -> Mux1/2  "<ve>"
  Bus Selector2/1 -> Mux1/1  "<vn>"
  Mux1/1 -> L1_Core/4(Vg)

== system Formation_FMS2/FMS Commander/Commander/Form_Subsystem/FormMission/FormMission_SubSystem ==
  FMS_In : Inport
  Reset : ResetPort  DisableCoverage=on
  Bus Assignment : BusAssignment  AssignedSignals=state,ax_cmd,ay_cmd,vh_cmd
  Compare To Constant : simulink/Logic and Bit Operations/Compare To Constant  relop===  const=1  OutDataTypeStr=boolean
  Constant : Constant  Value=0  OutDataTypeStr=Bus: FMS_Out_Bus
  Constant1 : Constant  Value=VehicleState.FormMission  OutDataTypeStr=Enum: VehicleState
  Constant2 : Constant  Value=uav_id  OutDataTypeStr=uint32
  Demux : Demux  Outputs=3
  Formation_Controller : Subsystem
  Leader_Controller : Subsystem
  Mux : Mux  Inputs=3
  Mux1 : Mux  Inputs=3
  Switch : Switch  Criteria=u2 ~= 0  Threshold=1  SaturateOnIntegerOverflow=off  InputSameDT=off
  FMS_Out : Outport  VectorParamsAs1DForOutWhenUnconnected=off
  wires:
  Constant/1 -> Bus Assignment/1
  Bus Assignment/1 -> FMS_Out/1
  Demux/1 -> Bus Assignment/3
  Demux/2 -> Bus Assignment/4
  Demux/3 -> Bus Assignment/5
  Constant1/1 -> Bus Assignment/2
  FMS_In/1 -> Formation_Controller/1(FMS_In), Leader_Controller/1(FMS_In)
  Leader_Controller/1(ax_cmd) -> Mux/1
  Leader_Controller/2(ay_cmd) -> Mux/2
  Leader_Controller/3(vh_cmd) -> Mux/3
  Formation_Controller/1(ux_cmd) -> Mux1/1
  Formation_Controller/2(uy_cmd) -> Mux1/2
  Formation_Controller/3(uz_cmd) -> Mux1/3
  Constant2/1 -> Compare To Constant/1
  Compare To Constant/1 -> Switch/2
  Mux/1 -> Switch/1
  Mux1/1 -> Switch/3
  Switch/1 -> Demux/1

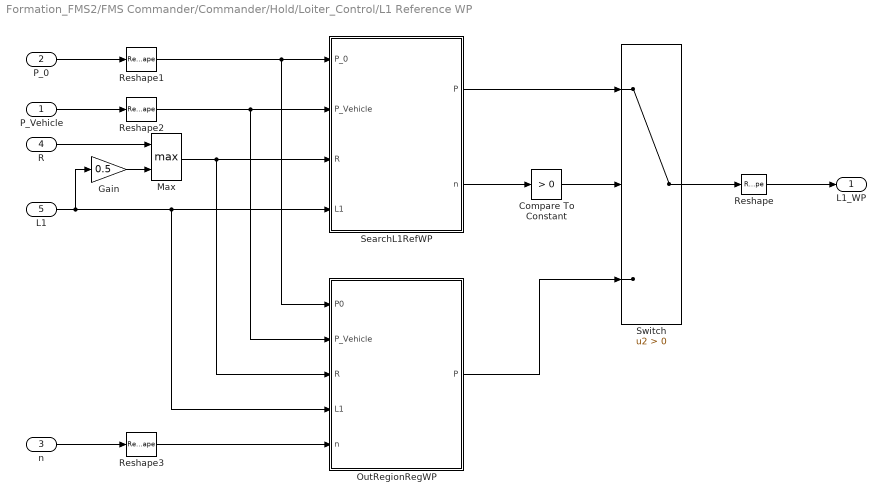
== system Formation_FMS2/FMS Commander/Commander/Hold/Loiter_Control/L1 Reference WP ==
  P_Vehicle : Inport
  P_0 : Inport  Port=2
  n : Inport  Port=3
  R : Inport  Port=4
  L1 : Inport  Port=5
  Compare To Constant : simulink/Logic and Bit Operations/Compare To Constant  relop=>  const=0  OutDataTypeStr=boolean
  Gain : Gain  Gain=0.5
  Max : MinMax  Function=max  Inputs=2
  OutRegionRegWP : MATLAB Function  TreatAsAtomicUnit=on
  Reshape : Reshape  OutputDimensionality=Customize  OutputDimensions=[2,1]
  Reshape1 : Reshape  OutputDimensionality=Column vector (2-D)
  Reshape2 : Reshape  OutputDimensionality=Column vector (2-D)
  Reshape3 : Reshape  OutputDimensionality=Column vector (2-D)
  SearchL1RefWP : MATLAB Function  TreatAsAtomicUnit=on
  Switch : Switch  Criteria=u2 > Threshold  SaturateOnIntegerOverflow=off  InputSameDT=off
  L1_WP : Outport  VectorParamsAs1DForOutWhenUnconnected=off
  wires:
  Reshape/1 -> L1_WP/1
  Compare To Constant/1 -> Switch/2
  SearchL1RefWP/2(n) -> Compare To Constant/1
  OutRegionRegWP/1(P) -> Switch/3
  Switch/1 -> Reshape/1
  SearchL1RefWP/1(P) -> Switch/1
  P_0/1 -> Reshape1/1
  P_Vehicle/1 -> Reshape2/1
  Max/1 -> OutRegionRegWP/3(R), SearchL1RefWP/3(R)
  L1/1 -> Gain/1, OutRegionRegWP/4(L1), SearchL1RefWP/4(L1)
  Reshape1/1 -> OutRegionRegWP/1(P0), SearchL1RefWP/1(P_0)
  Reshape2/1 -> OutRegionRegWP/2(P_Vehicle), SearchL1RefWP/2(P_Vehicle)
  n/1 -> Reshape3/1
  Reshape3/1 -> OutRegionRegWP/5(n)
  R/1 -> Max/1
  Gain/1 -> Max/2

== system Formation_FMS2/FMS Commander/Commander/Hold/Loiter_Control/L1_Core ==
  p_vehicle : Inport
  L1_WP : Inport  Port=2
  L1 : Inport  Port=3
  Vg : Inport  Port=4
  L1_Lateral_Acceleration : Subsystem
  Subtract : Sum  Inputs=+-
  ay_cmd_mPs2 : Outport  VectorParamsAs1DForOutWhenUnconnected=off
  wires:
  L1_WP/1 -> Subtract/1
  p_vehicle/1 -> Subtract/2
  L1/1 -> L1_Lateral_Acceleration/1(L1)
  Vg/1 -> L1_Lateral_Acceleration/2(Vg)
  Subtract/1 -> L1_Lateral_Acceleration/3(l1_path)
  L1_Lateral_Acceleration/1(l1_a_cmd) -> ay_cmd_mPs2/1

== system Formation_FMS2/FMS Commander/Commander/Hold/Loiter_Control/Reference_Point ==
  FMS_In : Inport
  Bus Selector1 : BusSelector  OutputSignals=Cmd_In.cur_waypoint
  Bus Selector2 : BusSelector  OutputSignals=INS_Out.vn,INS_Out.ve
  Bus Selector3 : BusSelector  OutputSignals=INS_Out.x_R,INS_Out.y_R
  Mux1 : Mux  Inputs=2
  Mux2 : Mux  Inputs=2
  Selector : Selector  InputPortWidth=3  IndexOptions=Index vector (dialog)  Indices=[1 2]  OutputSizes=1
  Vector Normalize : FC_Lib/Math/Vector Normalize
      settings: SourceProductName=Flight Control Toolbox
  start_vel : Delay  DelayLength=1  InitialConditionSource=Input port
      settings: InputPortMap=u0,p4
  p_vehicle : Outport  VectorParamsAs1DForOutWhenUnconnected=off
  p_0 : Outport  Port=2  VectorParamsAs1DForOutWhenUnconnected=off
  n : Outport  Port=3  VectorParamsAs1DForOutWhenUnconnected=off
  wires:
  Bus Selector2/2 -> Mux1/2  "<ve>"
  start_vel/1 -> Vector Normalize/1, start_vel/1
  Bus Selector2/1 -> Mux1/1  "<vn>"
  Vector Normalize/1 -> n/1
  FMS_In/1 -> Bus Selector3/1, Bus Selector2/1, Bus Selector1/1
  Mux1/1 -> start_vel/2
  Bus Selector3/1 -> Mux2/1  "<x_R>"
  Bus Selector3/2 -> Mux2/2  "<y_R>"
  Mux2/1 -> p_vehicle/1
  Bus Selector1/1 -> Selector/1  "<cur_waypoint>"
  Selector/1 -> p_0/1

== system Formation_FMS2/FMS Commander/Commander/Default/Loiter_Control/L1_Core/L1_Lateral_Acceleration ==
  L1 : Inport
  Vg : Inport  Port=2
  l1_path : Inport  Port=3
  Divide : Product  Inputs=*/
  Gain : Gain  Gain=2
  Included Angle : Subsystem
  Multiply1 : Product
  Saturation : Saturate  UpperLimit=pi/2  LowerLimit=-pi/2
  Sin : Trigonometry
  Square : Math  Operator=square  SignedPower=on
  Vector Modulus : FC_Lib/Math/Vector Modulus
      settings: SourceProductName=Flight Control Toolbox
  Vector Normalize : FC_Lib/Math/Vector Normalize
      settings: SourceProductName=Flight Control Toolbox
  Vector Normalize1 : FC_Lib/Math/Vector Normalize
      settings: SourceProductName=Flight Control Toolbox
  l1_a_cmd : Outport  VectorParamsAs1DForOutWhenUnconnected=off
  wires:
  Vector Modulus/1 -> Square/1
  L1/1 -> Divide/2
  Gain/1 -> Multiply1/2
  Square/1 -> Gain/1
  Vg/1 -> Vector Modulus/1, Vector Normalize/1
  Saturation/1 -> Sin/1
  l1_path/1 -> Vector Normalize1/1
  Sin/1 -> Multiply1/1  "sin_alpha"
  Vector Normalize1/1 -> Included Angle/2(vec2)
  Divide/1 -> l1_a_cmd/1  "l1_a_cmd"
  Multiply1/1 -> Divide/1
  Included Angle/1(angle_rad) -> Saturation/1  "L1_alpha"
  Vector Normalize/1 -> Included Angle/1(vec1)

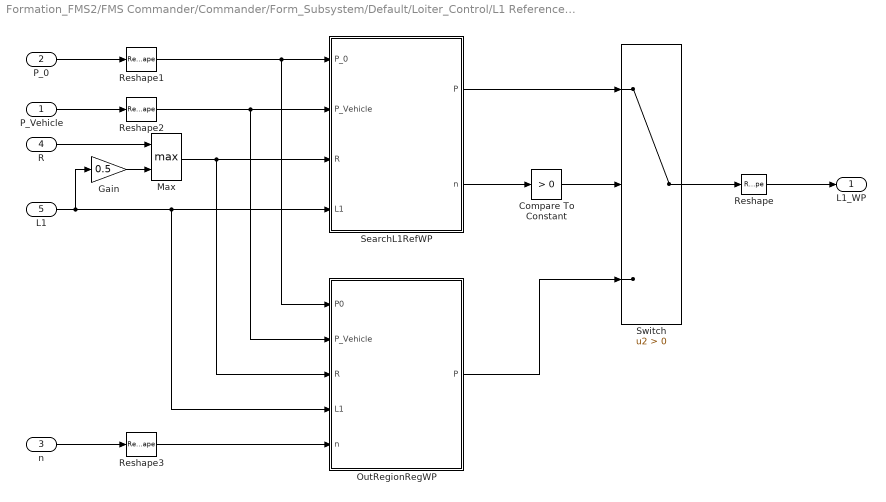
== system Formation_FMS2/FMS Commander/Commander/Form_Subsystem/Default/Loiter_Control/L1 Reference WP ==
  P_Vehicle : Inport
  P_0 : Inport  Port=2
  n : Inport  Port=3
  R : Inport  Port=4
  L1 : Inport  Port=5
  Compare To Constant : simulink/Logic and Bit Operations/Compare To Constant  relop=>  const=0  OutDataTypeStr=boolean
  Gain : Gain  Gain=0.5
  Max : MinMax  Function=max  Inputs=2
  OutRegionRegWP : MATLAB Function  TreatAsAtomicUnit=on
  Reshape : Reshape  OutputDimensionality=Customize  OutputDimensions=[2,1]
  Reshape1 : Reshape  OutputDimensionality=Column vector (2-D)
  Reshape2 : Reshape  OutputDimensionality=Column vector (2-D)
  Reshape3 : Reshape  OutputDimensionality=Column vector (2-D)
  SearchL1RefWP : MATLAB Function  TreatAsAtomicUnit=on
  Switch : Switch  Criteria=u2 > Threshold  SaturateOnIntegerOverflow=off  InputSameDT=off
  L1_WP : Outport  VectorParamsAs1DForOutWhenUnconnected=off
  wires:
  Gain/1 -> Max/2
  R/1 -> Max/1
  Reshape3/1 -> OutRegionRegWP/5(n)
  n/1 -> Reshape3/1
  Reshape2/1 -> SearchL1RefWP/2(P_Vehicle), OutRegionRegWP/2(P_Vehicle)
  Reshape1/1 -> SearchL1RefWP/1(P_0), OutRegionRegWP/1(P0)
  L1/1 -> SearchL1RefWP/4(L1), OutRegionRegWP/4(L1), Gain/1
  Max/1 -> SearchL1RefWP/3(R), OutRegionRegWP/3(R)
  P_Vehicle/1 -> Reshape2/1
  P_0/1 -> Reshape1/1
  SearchL1RefWP/1(P) -> Switch/1
  Switch/1 -> Reshape/1
  OutRegionRegWP/1(P) -> Switch/3
  SearchL1RefWP/2(n) -> Compare To Constant/1
  Compare To Constant/1 -> Switch/2
  Reshape/1 -> L1_WP/1

== system Formation_FMS2/FMS Commander/Commander/Form_Subsystem/Default/Loiter_Control/L1_Core ==
  p_vehicle : Inport
  L1_WP : Inport  Port=2
  L1 : Inport  Port=3
  Vg : Inport  Port=4
  L1_Lateral_Acceleration : Subsystem
  Subtract : Sum  Inputs=+-
  ay_cmd_mPs2 : Outport  VectorParamsAs1DForOutWhenUnconnected=off
  wires:
  L1_Lateral_Acceleration/1(l1_a_cmd) -> ay_cmd_mPs2/1
  Subtract/1 -> L1_Lateral_Acceleration/3(l1_path)
  Vg/1 -> L1_Lateral_Acceleration/2(Vg)
  L1/1 -> L1_Lateral_Acceleration/1(L1)
  p_vehicle/1 -> Subtract/2
  L1_WP/1 -> Subtract/1

== system Formation_FMS2/FMS Commander/Commander/Form_Subsystem/Default/Loiter_Control/Reference_Point ==
  FMS_In : Inport
  Bus Selector1 : BusSelector  OutputSignals=Cmd_In.cur_waypoint
  Bus Selector2 : BusSelector  OutputSignals=INS_Out.vn,INS_Out.ve
  Bus Selector3 : BusSelector  OutputSignals=INS_Out.x_R,INS_Out.y_R
  Mux1 : Mux  Inputs=2
  Mux2 : Mux  Inputs=2
  Selector : Selector  InputPortWidth=3  IndexOptions=Index vector (dialog)  Indices=[1 2]  OutputSizes=1
  Vector Normalize : FC_Lib/Math/Vector Normalize
      settings: SourceProductName=Flight Control Toolbox
  start_vel : Delay  DelayLength=1  InitialConditionSource=Input port
      settings: InputPortMap=u0,p4
  p_vehicle : Outport  VectorParamsAs1DForOutWhenUnconnected=off
  p_0 : Outport  Port=2  VectorParamsAs1DForOutWhenUnconnected=off
  n : Outport  Port=3  VectorParamsAs1DForOutWhenUnconnected=off
  wires:
  Selector/1 -> p_0/1
  Bus Selector1/1 -> Selector/1  "<cur_waypoint>"
  Mux2/1 -> p_vehicle/1
  Bus Selector3/2 -> Mux2/2  "<y_R>"
  Bus Selector3/1 -> Mux2/1  "<x_R>"
  Mux1/1 -> start_vel/2
  FMS_In/1 -> Bus Selector1/1, Bus Selector2/1, Bus Selector3/1
  Vector Normalize/1 -> n/1
  Bus Selector2/1 -> Mux1/1  "<vn>"
  start_vel/1 -> start_vel/1, Vector Normalize/1
  Bus Selector2/2 -> Mux1/2  "<ve>"

== system Formation_FMS2/FMS Commander/Commander/Form_Subsystem/FormAssemble/Mission_SubSystem/Airspeed Hold ==
  note: \mathrm{d}V_g = - \frac{V_g \times (1 + \mathrm{d}\tau)}{\tau}
  note: \tau _{left} = \frac{L*(1-R_{rem})}{V_g}
  FMS_In : Inport
  Bus Selector : BusSelector  OutputSignals=INS_Out.airspeed
  Bus Selector1 : BusSelector  Commented=on  OutputSignals=Formation_Cross.left_time
  Constant : Constant  Value=FMS_PARAM.FW_AIRSPD_TRIM
  Gain : Gain
  Gain1 : Gain  Commented=on  Gain=FORMATION_PARAM.ASSEMBLE_KT
  Sum : Sum  Inputs=-+|
  Sum1 : Sum  Inputs=++|
  Time Consensus Controller : MATLAB Function  Commented=on  TreatAsAtomicUnit=on  mask{uav_id=uav_id, adj_matrix=FORMATION_PARAM.ADJ_MARTIX}
  ax_cmd : Outport
  wires:
  Sum/1 -> Gain/1  "v_error"
  Gain/1 -> Sum1/2  "ax_cmd"
  Constant/1 -> Sum/2
  FMS_In/1 -> Bus Selector/1, Bus Selector1/1
  Bus Selector/1 -> Sum/1  "<airspeed>"
  Bus Selector1/1 -> Time Consensus Controller/1(left_time)  "<left_time>"
  Gain1/1 -> Sum1/1  "ax_cmd"
  Time Consensus Controller/1(ut_cmd) -> Gain1/1
  Sum1/1 -> ax_cmd/1

== system Formation_FMS2/FMS Commander/Commander/Form_Subsystem/FormAssemble/Mission_SubSystem/Altitude Control ==
  FMS_In : Inport
  Bus Selector3 : BusSelector  OutputSignals=INS_Out.h_R
  Gain : Gain  Gain=FMS_PARAM.Z_P
  Saturation1 : Saturate  UpperLimit=CONTROL_PARAM.FW_T_CLMB_MAX  LowerLimit=-CONTROL_PARAM.FW_T_SINK_MAX
  Sum2 : Sum  Inputs=|+-
  Target Height : Subsystem
  w_cmd_mPs : Outport  VectorParamsAs1DForOutWhenUnconnected=off
  wires:
  FMS_In/1 -> Bus Selector3/1, Target Height/1(FMS_In)
  Bus Selector3/1 -> Sum2/2  "<h_R>"
  Sum2/1 -> Gain/1
  Gain/1 -> Saturation1/1
  Target Height/1(h_R_sp) -> Sum2/1  "h_R_sp"
  Saturation1/1 -> w_cmd_mPs/1

== system Formation_FMS2/FMS Commander/Commander/Form_Subsystem/FormAssemble/Mission_SubSystem/Altitude_Hold ==
  FMS_In : Inport
  Bus Selector2 : BusSelector  OutputSignals=INS_Out.h_R
  Constant : Constant  Value=FMS_PARAM.FW_HEIGHT_TRIM
  Delay : Delay  DelayLength=1  InitialConditionSource=Input port
      settings: InputPortMap=u0,p4
  Gain2 : Gain  Gain=FMS_PARAM.Z_P  OutDataTypeStr=single
  Saturation : Saturate  UpperLimit=CONTROL_PARAM.FW_T_CLMB_MAX  LowerLimit=-CONTROL_PARAM.FW_T_SINK_MAX
  Sum : Sum  Inputs=-+|
  vh_cmd_mPs : Outport  VectorParamsAs1DForOutWhenUnconnected=off
  wires:
  Gain2/1 -> Saturation/1
  Bus Selector2/1 -> Sum/1  "<h_R>"
  Sum/1 -> Gain2/1  "h_err_R"
  Delay/1 -> Sum/2, Delay/1  "h_cmd_R"
  FMS_In/1 -> Bus Selector2/1
  Saturation/1 -> vh_cmd_mPs/1
  Constant/1 -> Delay/2

== system Formation_FMS2/FMS Commander/Commander/Form_Subsystem/FormAssemble/Mission_SubSystem/Position Command ==
  FMS_In : Inport
  L1 Control : Subsystem
  WayPoints : Subsystem
  ay_cmd_mPs2 : Outport  VectorParamsAs1DForOutWhenUnconnected=off
  wires:
  FMS_In/1 -> L1 Control/4(FMS_In), WayPoints/1(FMS_In)
  WayPoints/2(p2) -> L1 Control/2(p2)
  WayPoints/3(p3) -> L1 Control/3(p3)
  WayPoints/1(p1) -> L1 Control/1(p1)
  L1 Control/1(ay_cmd_mPs2) -> ay_cmd_mPs2/1

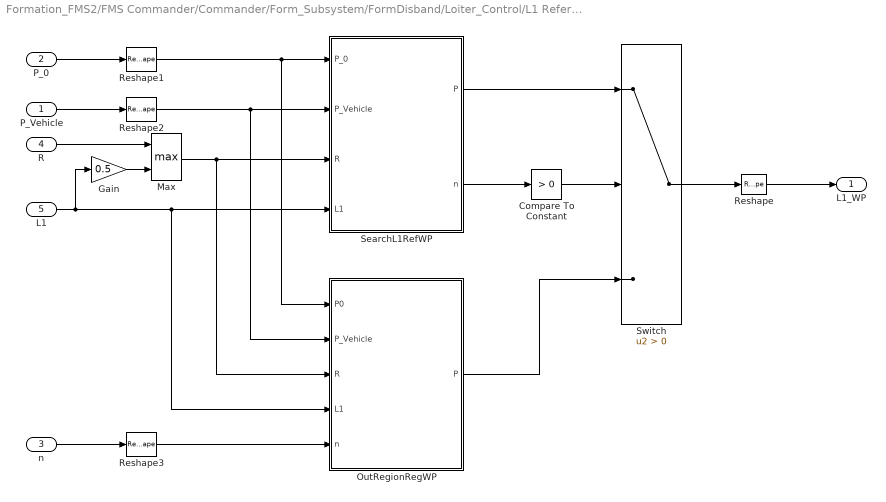
== system Formation_FMS2/FMS Commander/Commander/Form_Subsystem/FormDisband/Loiter_Control/L1 Reference WP ==
  P_Vehicle : Inport
  P_0 : Inport  Port=2
  n : Inport  Port=3
  R : Inport  Port=4
  L1 : Inport  Port=5
  Compare To Constant : simulink/Logic and Bit Operations/Compare To Constant  relop=>  const=0  OutDataTypeStr=boolean
  Gain : Gain  Gain=0.5
  Max : MinMax  Function=max  Inputs=2
  OutRegionRegWP : MATLAB Function  TreatAsAtomicUnit=on
  Reshape : Reshape  OutputDimensionality=Customize  OutputDimensions=[2,1]
  Reshape1 : Reshape  OutputDimensionality=Column vector (2-D)
  Reshape2 : Reshape  OutputDimensionality=Column vector (2-D)
  Reshape3 : Reshape  OutputDimensionality=Column vector (2-D)
  SearchL1RefWP : MATLAB Function  TreatAsAtomicUnit=on
  Switch : Switch  Criteria=u2 > Threshold  SaturateOnIntegerOverflow=off  InputSameDT=off
  L1_WP : Outport  VectorParamsAs1DForOutWhenUnconnected=off
  wires:
  Gain/1 -> Max/2
  R/1 -> Max/1
  Reshape3/1 -> OutRegionRegWP/5(n)
  n/1 -> Reshape3/1
  Reshape2/1 -> SearchL1RefWP/2(P_Vehicle), OutRegionRegWP/2(P_Vehicle)
  Reshape1/1 -> SearchL1RefWP/1(P_0), OutRegionRegWP/1(P0)
  L1/1 -> SearchL1RefWP/4(L1), OutRegionRegWP/4(L1), Gain/1
  Max/1 -> SearchL1RefWP/3(R), OutRegionRegWP/3(R)
  P_Vehicle/1 -> Reshape2/1
  P_0/1 -> Reshape1/1
  SearchL1RefWP/1(P) -> Switch/1
  Switch/1 -> Reshape/1
  OutRegionRegWP/1(P) -> Switch/3
  SearchL1RefWP/2(n) -> Compare To Constant/1
  Compare To Constant/1 -> Switch/2
  Reshape/1 -> L1_WP/1

== system Formation_FMS2/FMS Commander/Commander/Form_Subsystem/FormDisband/Loiter_Control/L1_Core ==
  p_vehicle : Inport
  L1_WP : Inport  Port=2
  L1 : Inport  Port=3
  Vg : Inport  Port=4
  L1_Lateral_Acceleration : Subsystem
  Subtract : Sum  Inputs=+-
  ay_cmd_mPs2 : Outport  VectorParamsAs1DForOutWhenUnconnected=off
  wires:
  L1_Lateral_Acceleration/1(l1_a_cmd) -> ay_cmd_mPs2/1
  Subtract/1 -> L1_Lateral_Acceleration/3(l1_path)
  Vg/1 -> L1_Lateral_Acceleration/2(Vg)
  L1/1 -> L1_Lateral_Acceleration/1(L1)
  p_vehicle/1 -> Subtract/2
  L1_WP/1 -> Subtract/1

== system Formation_FMS2/FMS Commander/Commander/Form_Subsystem/FormDisband/Loiter_Control/Reference_Point ==
  FMS_In : Inport
  Bus Selector1 : BusSelector  OutputSignals=Cmd_In.cur_waypoint
  Bus Selector2 : BusSelector  OutputSignals=INS_Out.vn,INS_Out.ve
  Bus Selector3 : BusSelector  OutputSignals=INS_Out.x_R,INS_Out.y_R
  Mux1 : Mux  Inputs=2
  Mux2 : Mux  Inputs=2
  Selector : Selector  InputPortWidth=3  IndexOptions=Index vector (dialog)  Indices=[1 2]  OutputSizes=1
  Vector Normalize : FC_Lib/Math/Vector Normalize
      settings: SourceProductName=Flight Control Toolbox
  start_vel : Delay  DelayLength=1  InitialConditionSource=Input port
      settings: InputPortMap=u0,p4
  p_vehicle : Outport  VectorParamsAs1DForOutWhenUnconnected=off
  p_0 : Outport  Port=2  VectorParamsAs1DForOutWhenUnconnected=off
  n : Outport  Port=3  VectorParamsAs1DForOutWhenUnconnected=off
  wires:
  Selector/1 -> p_0/1
  Bus Selector1/1 -> Selector/1  "<cur_waypoint>"
  Mux2/1 -> p_vehicle/1
  Bus Selector3/2 -> Mux2/2  "<y_R>"
  Bus Selector3/1 -> Mux2/1  "<x_R>"
  Mux1/1 -> start_vel/2
  FMS_In/1 -> Bus Selector1/1, Bus Selector2/1, Bus Selector3/1
  Vector Normalize/1 -> n/1
  Bus Selector2/1 -> Mux1/1  "<vn>"
  start_vel/1 -> start_vel/1, Vector Normalize/1
  Bus Selector2/2 -> Mux1/2  "<ve>"
